simulink model "Osservatore"  (R2023a)
settings: Solver=VariableStepAuto  StartTime=0.0  StopTime=15  RelTol=1e-3
undefined symbols (not defined in the file or in its folder): A, B, C, L
settings Model: Creator=vince  LastModifiedBy=vince

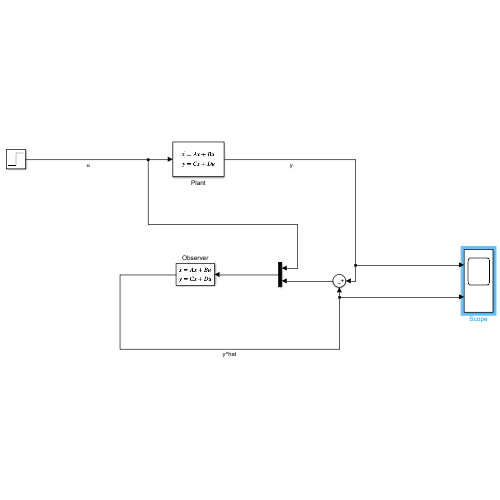
[thumbnail: Simulink's stored preview of the top-level diagram]
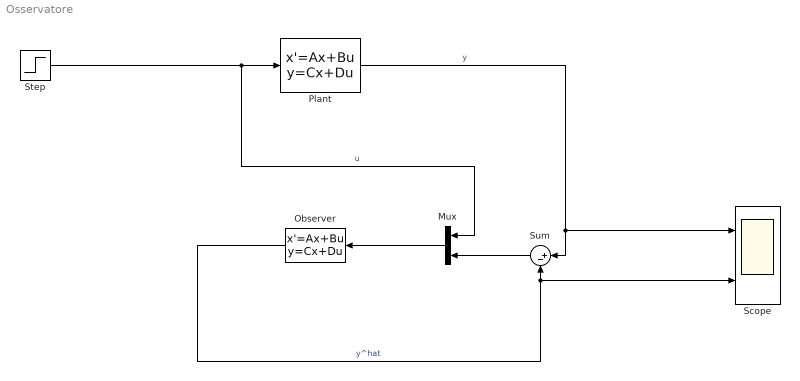
== system Osservatore ==
  Mux : Mux  Inputs=2
  Observer : StateSpace  A=A  B=[B L]  C=C  D=[0 0]  InitialCondition=0
  Plant : StateSpace  A=A  B=B  C=C  D=[0]  InitialCondition=[1 3]
  Scope : Scope  NumInputPorts=2
  Step : Step  Time=0  SampleTime=0
  Sum : Sum  Inputs=|+-
  wires:
  Mux/1 -> Observer/1
  Step/1 -> Plant/1, Mux/1  "u"
  Plant/1 -> Sum/1, Scope/1  "y"
  Observer/1 -> Scope/2, Sum/2  "y^hat"
  Sum/1 -> Mux/2
